simulink model "ARCH_MAX_DS3231"  (R2015a)
settings: Solver=FixedStepDiscrete  SolverMode=SingleTasking  StartTime=0.0  StopTime=10.0  FixedStep=1e-3  RelTol=1e-3
libraries: mbed_lib x4, mbed_i2c_several x1
settings Model: Creator=oh  LastModifiedBy=Stuv
settings OptimizationCC: OptimizeModelRefInitCode=on  LifeSpan=1
settings HardwareCC: ProdLargestAtomicInteger=Long  ProdLargestAtomicFloat=Double  ProdEndianess=LittleEndian  ProdHWDeviceType=ARM Compatible->ARM Cortex
settings RTWCC: SystemTargetFile=mbed.tlc  TemplateMakefile=mbed.tmf  Description=Mbed Target (Embedded Target)  TargetLang=C++
settings CodeAppCC: IgnoreCustomStorageClasses=off
settings STFCustomTargetCC: CombineOutputUpdateFcns=on  SupportContinuousTime=off  SupportVariableSizeSignals=off  SystemTargetFile=mbed.tlc
settings ERTTargetCC: SupportContinuousTime=off  SupportVariableSizeSignals=off  ERTCustomFileTemplate=mbed_file_process.tlc

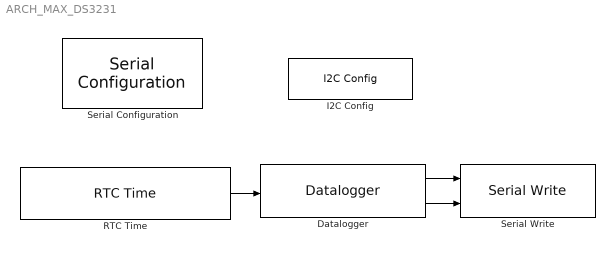
== system ARCH_MAX_DS3231 ==
  Datalogger : mbed_lib/Utilities/Datalogger  TypeInputPorts={ 'uint32' 1 }  TypeOfInputs={'1*uint32'}  BufferSize=100  errEn=off  SampleTime=-1
  I2C Config : mbed_lib/I2C/I2C Config  Priority=0  I2cPort=1  SParameter6=100000  SParameter2=B  SParameter3=9  SParameter4=B  SParameter5=8
  RTC Time : mbed_i2c_several/RTC Time  SampleTime=1  i2cbus=1
  Serial Configuration : mbed_lib/Serial/Serial Configuration  SerialPort=1  TXPort=C  TXPin=6  RXPort=C  RXPin=7  BaudRate=9600
  Serial Write : mbed_lib/Serial/Serial Write  SerialPort=1  numData=on  SampleTime=-1
  wires:
  RTC Time/1 -> Datalogger/1
  Datalogger/1 -> Serial Write/1
  Datalogger/2 -> Serial Write/2
